simulink subsystem "motores"  (R2023b)
settings: Solver=VariableStepAuto  StartTime=0.0  StopTime=10.0  RelTol=1e-3
settings Model: Creator=Diego  LastModifiedBy=Diego

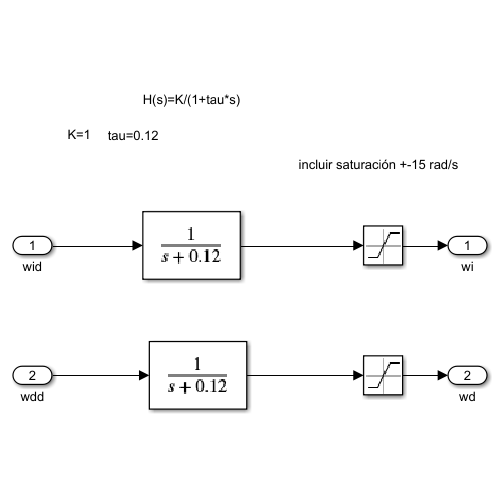
[thumbnail: Simulink's stored preview of the top-level diagram]
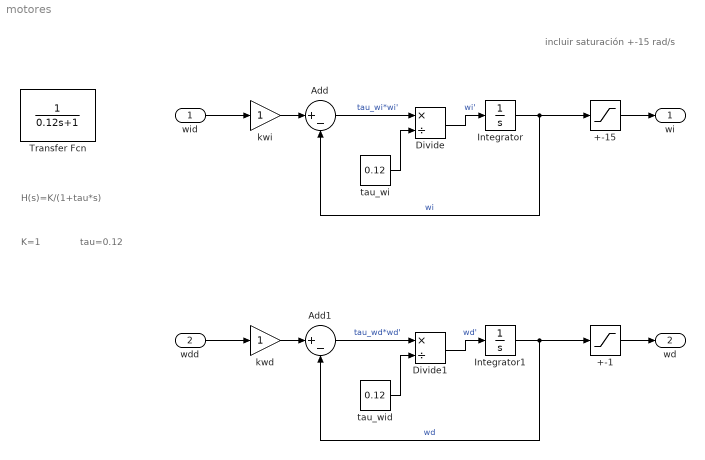
== system motores ==
  note: H(s)=K/(1+tau*s)
  note: K=1
  note: tau=0.12
  note: incluir saturación +-15 rad/s
  wid : Inport
  wdd : Inport  Port=2
  +-1 : Saturate  UpperLimit=15  LowerLimit=-15
  +-15 : Saturate  UpperLimit=15  LowerLimit=-15
  Add : Sum  Inputs=|+-
  Add1 : Sum  Inputs=|+-
  Divide : Product  Inputs=*/
  Divide1 : Product  Inputs=*/
  Integrator : Integrator
  Integrator1 : Integrator
  Transfer Fcn : TransferFcn  Denominator=[0.12 1]
  kwd : Gain
  kwi : Gain
  tau_wi : Constant  Value=0.12
  tau_wid : Constant  Value=0.12
  wi : Outport
  wd : Outport  Port=2
  wires:
  +-1/1 -> wd/1
  +-15/1 -> wi/1
  wid/1 -> kwi/1
  kwi/1 -> Add/1
  Integrator/1 -> Add/2, +-15/1  "wi"
  Add/1 -> Divide/1  "tau_wi*wi'"
  Divide/1 -> Integrator/1  "wi'"
  tau_wi/1 -> Divide/2
  kwd/1 -> Add1/1
  Divide1/1 -> Integrator1/1  "wd'"
  Integrator1/1 -> Add1/2, +-1/1  "wd"
  wdd/1 -> kwd/1
  tau_wid/1 -> Divide1/2
  Add1/1 -> Divide1/1  "tau_wd*wd'"
